simulink model "DotFinder_th"  (R2018b)
settings: Solver=FixedStepAuto  StartTime=0.0  StopTime=0  FixedStep=1  RelTol=1e-3
StopFcn:
  | imshow(image.signals.values)
undefined symbols (not defined in the file or in its folder): Rec, SDTV
libraries: visionconversions x1, dotFinder_ul x1, visionsources x1
settings Model: Creator=mcobb  LastModifiedBy=mcobb
settings DebuggingCC: LibraryContextMissingDiagnostic=none
settings SFSimCC: SimUseLocalCustomCode=off
settings RTWCC: RTWUseLocalCustomCode=off

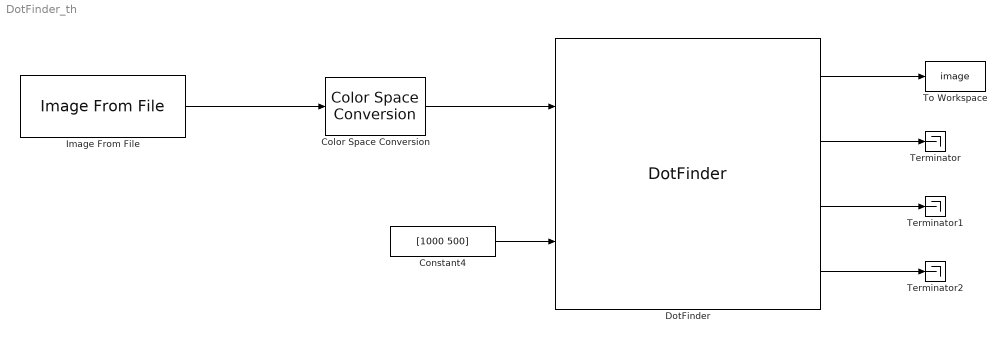
== system DotFinder_th ==
  Color Space Conversion : visionconversions/Color Space  Conversion  conversion=Obsolete  conversionActive=R'G'B' to intensity  wp_str=D65  rec=Rec. 601 (SDTV)  sys=1125/60/2:1  imagePorts=One multidimensional signal
      settings: SourceProductName=Computer Vision System Toolbox
  Constant4 : Constant  Value=[1000 500]
  DotFinder : dotFinder_ul/DotFinder  ROIPositionHoldEnable=on  ROIPositionHoldCoordinates=[275 650]  ROIDimVec_px=[90 60]  ROIHalfDimVec_px=[45 30]  ROISplitDims_px=[1 90 ; 1 30 ; 1 90 ; 31 29]  DotOrientation=Horizontal  OverlayOutput=on  ImageDimensions=[765 998]  CrosshairPixelWidth_px=1
  Image From File : visionsources/Image From File  Tag=vipblks_nd  FileName=C:\Users\mcobb\Google Drive\speedgoatTest\test4\testImage.PNG  imagePorts=One multidimensional signal  Ts=inf  ImageDataType=Inherit from input image  Signed=on  WordLength=16  sdImageDataType=uint(8)  FractionLengthMode=User-defined  FractionLength=15  OutPortLabels=R|G|B
      settings: SourceProductName=Computer Vision System Toolbox
  Terminator : Terminator
  Terminator1 : Terminator
  Terminator2 : Terminator
  To Workspace : ToWorkspace  VariableName=image  SaveFormat=Structure With Time  SampleTime=-1
  wires:
  Image From File/1 -> Color Space Conversion/1
  Color Space Conversion/1 -> DotFinder/1
  Constant4/1 -> DotFinder/2
  DotFinder/1 -> To Workspace/1
  DotFinder/2 -> Terminator/1
  DotFinder/3 -> Terminator1/1
  DotFinder/4 -> Terminator2/1
